simulink model "CLA_Sample"  (R2022b)
settings: Solver=FixedStepAuto  StartTime=0.0  StopTime=Inf  RelTol=1e-3  EnableMultiTasking=on
model workspace (MAT data in the model file):
  ADC_Gain = 1241.21212121
  DAC_Gain = 0.000805860805861
  Inductor_Current_Divider_Gain_Phase_A = 33.4
  Inductor_Current_Divider_Gain_Phase_B = 33.4
  Vbulk_Divider_Gain = 276.854928018
  Vin_Divider_Gain = 556.17352614
undefined symbols (not defined in the file or in its folder): GPTRIP1SEL, GPTRIP2SEL, SCI_A_Transmit, SCI_A_Transmit_Current_Suffix, SCI_A_Transmit_one_shot_Suffix, SCI_A_Transmit_Polarity_Suffix, SCI_A_Transmit_relay_Suffix, SCI_A_Transmit_Vbulk_Suffix, SCI_A_Transmit_Vin_rms_Suffix, SCI_A_Transmit_Vin_Suffix, SCI_A_Transmit_Vmid_Suffix, SCI_A_Transmit_Vp_Suffix, SCI_A_Transmit_Vpfc_Suffix, TZ1, TZ2
libraries: c280xlib x33, simulink x17, c2802xlib x15, c2000lib x1, c2806xlib x1
(part 5 of 5)

== system CLA_Sample/PWM Update @65KHz/Fixed Duty update_Phase_B/Archive/If Action Subsystem3/If Action Subsystem5 ==
  Action Port : ActionPort
  Constant : Constant  Value=100
  Data Store Read : DataStoreRead  DataStoreName=PWM_Duty_UART  IndexOptions=Index vector (dialog)  Indices=1  OutputSizes=1
  Data Store Read2 : DataStoreRead  DataStoreName=PWM_Duty_UART  IndexOptions=Index vector (dialog)  Indices=1  OutputSizes=1
  Data Store Read3 : DataStoreRead  DataStoreName=PFC_en_Phase_A  IndexOptions=Index vector (dialog)  Indices=1  OutputSizes=1
  Data Store Read4 : DataStoreRead  DataStoreName=One_Shot_Bar  IndexOptions=Index vector (dialog)  Indices=1  OutputSizes=1
  Data Store Write : DataStoreWrite  DataStoreName=PWM_DutyNearzero  IndexOptions=Index vector (dialog)  Indices=1  OutputSizes=1
  Product1 : Product  Inputs=3  OutDataTypeStr=double
  Subtract : Sum  Inputs=+-
  wires:
  Data Store Read4/1 -> Product1/2
  Data Store Read3/1 -> Product1/1
  Data Store Read2/1 -> Product1/3
  Constant/1 -> Subtract/1
  Data Store Read/1 -> Subtract/2
  Product1/1 -> Data Store Write/1

== system CLA_Sample/PWM Update @65KHz/Fixed Duty update_Phase_C/Archive/If Action Subsystem3/If Action Subsystem4 ==
  Action Port : ActionPort
  Data Store Read : DataStoreRead  DataStoreName=PWM_Duty_UART  IndexOptions=Index vector (dialog)  Indices=1  OutputSizes=1
  Data Store Read2 : DataStoreRead  DataStoreName=PWM_Duty_UART  IndexOptions=Index vector (dialog)  Indices=1  OutputSizes=1
  Data Store Read3 : DataStoreRead  DataStoreName=PFC_en_Phase_A  IndexOptions=Index vector (dialog)  Indices=1  OutputSizes=1
  Data Store Read4 : DataStoreRead  DataStoreName=One_Shot_Bar  IndexOptions=Index vector (dialog)  Indices=1  OutputSizes=1
  Data Store Write : DataStoreWrite  DataStoreName=PWM_DutyNearzero  IndexOptions=Index vector (dialog)  Indices=1  OutputSizes=1
  Product1 : Product  Inputs=3  OutDataTypeStr=double
  wires:
  Product1/1 -> Data Store Write/1
  Data Store Read3/1 -> Product1/1
  Data Store Read4/1 -> Product1/2
  Data Store Read2/1 -> Product1/3

== system CLA_Sample/PWM Update @65KHz/Fixed Duty update_Phase_C/Archive/If Action Subsystem3/If Action Subsystem5 ==
  Action Port : ActionPort
  Constant : Constant  Value=100
  Data Store Read : DataStoreRead  DataStoreName=PWM_Duty_UART  IndexOptions=Index vector (dialog)  Indices=1  OutputSizes=1
  Data Store Read2 : DataStoreRead  DataStoreName=PWM_Duty_UART  IndexOptions=Index vector (dialog)  Indices=1  OutputSizes=1
  Data Store Read3 : DataStoreRead  DataStoreName=PFC_en_Phase_A  IndexOptions=Index vector (dialog)  Indices=1  OutputSizes=1
  Data Store Read4 : DataStoreRead  DataStoreName=One_Shot_Bar  IndexOptions=Index vector (dialog)  Indices=1  OutputSizes=1
  Data Store Write : DataStoreWrite  DataStoreName=PWM_DutyNearzero  IndexOptions=Index vector (dialog)  Indices=1  OutputSizes=1
  Product1 : Product  Inputs=3  OutDataTypeStr=double
  Subtract : Sum  Inputs=+-
  wires:
  Data Store Read4/1 -> Product1/2
  Data Store Read3/1 -> Product1/1
  Data Store Read2/1 -> Product1/3
  Constant/1 -> Subtract/1
  Data Store Read/1 -> Subtract/2
  Product1/1 -> Data Store Write/1

== stateflow chart CLA_Sample/Calibration,RMS, Fault Protection @5kHz/Fault checking/If Action Subsystem/Phase_C_Fault/Fault Check (Input OVP)_Phase_C/Chart1 ==
  (default) -> (junction 2)
  (junction 2) -> (junction 81) [order 1] : [input > Voff_Threshold]
  (junction 81) -> (junction 82) : {
      | Input_OVP_Flag=1;
      | Voff_Threshold=95;
      | }
  (junction 2) -> (junction 84) [order 2] : {
      | Input_OVP_Flag=0;
      | Voff_Threshold = 100;
      | }
  (junction 82) -> (junction 84)
  data: input input double; Input_OVP_Flag output double =0; Voff_Threshold local =100

== stateflow chart CLA_Sample/Calibration,RMS, Fault Protection @5kHz/Fault checking/If Action Subsystem/Phase_C_Fault/Fault Check (Input UVP)_Phase_C/Chart1 ==
  (default) -> (junction 2)
  (junction 2) -> (junction 81) [order 1] : [input > Von_Threshold]
  (junction 81) -> (junction 82) : {
      | Input_UVP_Flag=0;
      | Von_Threshold=8;
      | }
  (junction 2) -> (junction 84) [order 2] : {
      | Input_UVP_Flag=1;
      | Von_Threshold = 12;
      | }
  (junction 82) -> (junction 84)
  data: input input double; Input_UVP_Flag output double =1; Von_Threshold local =12

== stateflow chart CLA_Sample/Calibration,RMS, Fault Protection @5kHz/Fault checking/If Action Subsystem/Phase_C_Fault/Input current_OCP_Phase_C/Chart2 ==
  note: Input_in > 1A, Iin_OCP_Flag=1.
  (default) -> (junction 2)
  (junction 2) -> (junction 81) [order 1] : [input_Iin > OCP_Threshold]
  (junction 81) -> (junction 82) : {Iin_OCP_Flag=1;
      | OCP_Threshold=14;
      | }
  (junction 2) -> (junction 84) [order 2] : {Iin_OCP_Flag=0;
      | OCP_Threshold=15;}
  (junction 82) -> (junction 84)
  data: input_Iin input double; Iin_OCP_Flag output double =1; data local; OCP_Threshold input; OCP_Threshold output

== stateflow chart CLA_Sample/Calibration,RMS, Fault Protection @5kHz/Fault checking/If Action Subsystem/PFC_en_update_Phase_C/Chart ==
  note: Local variables
      | VbusRefTemp
      | SoftStartCnt
  note: Verror = Vbulk_Ref_ADC_adjusted - Vbulk_ADC;
  (default) -> (junction 47)
  (junction 47) -> (junction 50) [order 4]
  (junction 47) -> (junction 68) [order 1] : [Vin_OVP_Flag]
  (junction 68) -> (junction 80) : {PFC_en=0;}
  (junction 47) -> (junction 15) [order 2] : [Iin_OCP_Flag]
  (junction 50) -> (junction 52) : {
      | PFC_en=1;
      | PFC_en1=1;
      | }
  (junction 47) -> (junction 5) [order 3] : [Vin_UVP_Flag]
  (junction 80) -> (junction 82)
  (junction 82) -> (junction 84)
  (junction 5) -> (junction 38) : {
      | PFC_en=0;
      | PFC_en1=0;
      | }
  (junction 15) -> (junction 20) : {PFC_en=0;
      | PFC_en1=0;}
  (junction 52) -> (junction 38)
  (junction 20) -> (junction 38)
  (junction 84) -> (junction 20)
  data: Vin_UVP_Flag input; VbusRefTemp local =0; Vin_OVP_Flag input; SoftStartCnt local =0; Vbulk_Ref_ADC_Hard_Value local =0; UVPCnt local =0; PFC_en output; PFC_en1 output; Iin_OCP_Flag input; Iin_OCP_Flag1 local

== stateflow chart CLA_Sample/Calibration,RMS, Fault Protection @5kHz/Polarity & Near Zero check/Polarity_Near_zero_Phase_C/Chart ==
  note: 1-> Polarity -> Positive Half cycle
      | 0-> Polarity -> Negative Half cycle
  (default) -> (junction 89) : {Vabs=abs(input);}
  (junction 89) -> (junction 99) [order 1] : [input>Vref]
  (junction 89) -> (junction 103) [order 2] : {Polarity=0;}
  (junction 99) -> (junction 101) : {Polarity=1;}
  (junction 103) -> (junction 142) [order 3]
  (junction 101) -> (junction 103)
  (junction 103) -> (junction 133) [order 1] : [Near_zero==0]
      | {Count = Count+1;}
  (junction 142) -> (junction 146)
  (junction 103) -> (junction 120) [order 2] : [Vabs<VZCD_Gap]
      | {Near_zero=0;}
  (junction 133) -> (junction 120) [order 2]
  (junction 133) -> (junction 136) [order 1] : [Count>10]
      | {Near_zero=1;
      | Count=0;}
  (junction 146) -> (junction 120)
  (junction 136) -> (junction 120)
  data: input input double; Polarity output; Vabs local double =0; Vref input; VZCD_Gap input; Near_zero output double =0; Count local =0

== stateflow chart CLA_Sample/Calibration,RMS, Fault Protection @5kHz/Voltage RMS//Averag Calculation/Phase_C/RMS Current Calculation_Phase_C/Chart ==
  note: counter > (0.5 / minimum line frequncy) x execution frequency of this loop
      | = [ 1 / (2 x 47 Hz) ] x 5 kHz = 53.191
      | Minimum frequency detection is 47Hz.
      | This can detect the voltage change in ~10.63 ms (max).
  (default) -> (junction 2) : {Vabs=abs(input);}
  (junction 2) -> (junction 81) [order 1] : [Vabs>max_tmp]
  (junction 81) -> (junction 82) : {
      | max_tmp=Vabs;
      | counter=counter+1;
      | timer=timer+1;
      | }
  (junction 2) -> (junction 84) [order 2] : {
      | counter=counter+1;
      | timer=timer+1;
      | }
  (junction 82) -> (junction 84)
  (junction 84) -> (junction 8)
  (junction 8) -> (junction 71) [order 1] : [counter==53]
  (junction 71) -> (junction 72) : {
      | counter=0;
      | Vpeak=max_tmp;
      | Vrms = 0.7071*Vpeak;
      | max_tmp=0;
      | }
  (junction 8) -> (junction 64) [order 2]
  (junction 72) -> (junction 64)
  data: input input double; max_tmp local double =0; counter local double =0; Vpeak output; Vrms output; timer local double =0; Vabs local double =0

== stateflow chart CLA_Sample/Calibration,RMS, Fault Protection @5kHz/Voltage RMS//Averag Calculation/Phase_A/RMS Current Calculation_Phase_A/Chart ==
  note: counter > (0.5 / minimum line frequncy) x execution frequency of this loop
      | = [ 1 / (2 x 47 Hz) ] x 5 kHz = 53.191
      | Minimum frequency detection is 47Hz.
      | This can detect the voltage change in ~10.63 ms (max).
  (default) -> (junction 2) : {Vabs=abs(input);}
  (junction 2) -> (junction 81) [order 1] : [Vabs>max_tmp]
  (junction 81) -> (junction 82) : {
      | max_tmp=Vabs;
      | counter=counter+1;
      | timer=timer+1;
      | }
  (junction 2) -> (junction 84) [order 2] : {
      | counter=counter+1;
      | timer=timer+1;
      | }
  (junction 82) -> (junction 84)
  (junction 84) -> (junction 8)
  (junction 8) -> (junction 71) [order 1] : [counter==53]
  (junction 71) -> (junction 72) : {
      | counter=0;
      | Vpeak=max_tmp;
      | Vrms = 0.7071*Vpeak;
      | max_tmp=0;
      | }
  (junction 8) -> (junction 64) [order 2]
  (junction 72) -> (junction 64)
  data: input input double; max_tmp local double =0; counter local double =0; Vpeak output; Vrms output; timer local double =0; Vabs local double =0

== stateflow chart CLA_Sample/Calibration,RMS, Fault Protection @5kHz/Voltage RMS//Averag Calculation/Phase_B/RMS Current Calculation_Phase_B/Chart ==
  note: counter > (0.5 / minimum line frequncy) x execution frequency of this loop
      | = [ 1 / (2 x 47 Hz) ] x 5 kHz = 53.191
      | Minimum frequency detection is 47Hz.
      | This can detect the voltage change in ~10.63 ms (max).
  (default) -> (junction 2) : {Vabs=abs(input);}
  (junction 2) -> (junction 81) [order 1] : [Vabs>max_tmp]
  (junction 81) -> (junction 82) : {
      | max_tmp=Vabs;
      | counter=counter+1;
      | timer=timer+1;
      | }
  (junction 2) -> (junction 84) [order 2] : {
      | counter=counter+1;
      | timer=timer+1;
      | }
  (junction 82) -> (junction 84)
  (junction 84) -> (junction 8)
  (junction 8) -> (junction 71) [order 1] : [counter==53]
  (junction 71) -> (junction 72) : {
      | counter=0;
      | Vpeak=max_tmp;
      | Vrms = 0.7071*Vpeak;
      | max_tmp=0;
      | }
  (junction 8) -> (junction 64) [order 2]
  (junction 72) -> (junction 64)
  data: input input double; max_tmp local double =0; counter local double =0; Vpeak output; Vrms output; timer local double =0; Vabs local double =0

== stateflow chart CLA_Sample/PWM Update @65KHz/Closed loop PWM generation (Control)/If Action Subsystem/Function-Call Subsystem/Chart4 ==
  (default) -> (junction 18) : {
      | output_y = b0*input_u + b1*input_z1 + b2*input_z2 - a1*output_z1 - a2*output_z2;
      |
      | }
  (junction 18) -> (junction 23) [commented out]
  (junction 18) -> (junction 15) [order 2]
  (junction 18) -> (junction 15) [order 1] : [output_y>Max_Duty]{output_y=Max_Duty;}
  (junction 23) -> (junction 27) [commented out] : [output_y<23]
      |
      | {
      | output_y=0;
      | }
  (junction 27) -> (junction 15) [commented out]
  (junction 15) -> (junction 16) : {
      | input_z2 = input_z1;
      | input_z1 = input_u;
      | output_z2 = output_z1;
      | output_z1 = output_y;}
  (junction 16) -> (junction 31) [order 2]
  (junction 16) -> (junction 31) [order 1] : [output_y<45]
      | {
      | output_y=0;
      | }
  data: Max_Duty input; input_z2 local =0; input_z1 local =0; output_z2 local =0; output_z1 local =0; output_y output; input_u input; b0 input; b1 input; b2 input; a1 input; a2 input

== stateflow chart CLA_Sample/Calibration,RMS, Fault Protection @5kHz/Calibration/Calibration_3phase/Chart ==
  note: Local variables
      | VbusRefTemp
      | SoftStartCnt
  note: Verror = Vbulk_Ref_ADC_adjusted - Vbulk_ADC;
  (default) -> (junction 47)
  (junction 47) -> (junction 50) [order 4]
  (junction 47) -> (junction 68) [order 1] : [~Calibration_Done_Phase_C]
  (junction 68) -> (junction 80) : {Calibration_Done=0;}
  (junction 47) -> (junction 15) [order 2] : [~Calibration_Done_Phase_B]
  (junction 50) -> (junction 52) : {
      | Calibration_Done=1;
      | }
  (junction 47) -> (junction 5) [order 3] : [~Calibration_Done_Phase_A]
  (junction 80) -> (junction 82)
  (junction 82) -> (junction 84)
  (junction 5) -> (junction 38) : {
      | Calibration_Done=0;
      | }
  (junction 15) -> (junction 20) : {Calibration_Done=0;}
  (junction 52) -> (junction 38)
  (junction 20) -> (junction 38)
  (junction 84) -> (junction 20)
  data: Calibration_Done_Phase_A input; Calibration_Done_Phase_B input; VbusRefTemp local =0; SoftStartCnt local =0; Vbulk_Ref_ADC_Hard_Value local =0; UVPCnt local =0; Calibration_Done output; Calibration_Done_Phase_C input; Iin_OCP_Flag1 local

== stateflow chart CLA_Sample/Calibration,RMS, Fault Protection @5kHz/Fault checking/If Action Subsystem/Output Voltage_Latch_OVP/Chart2 ==
  note: "One_Shot_Bar = 0" means fault occurs and turn off switching.
  (default) -> (junction 2)
  (junction 2) -> (junction 81) [order 1] : [input_Vbulk > Vbulk_OVP_Threshold]
  (junction 81) -> (junction 82) : {
      | One_Shot_Bar=0;
      | }
  (junction 2) -> (junction 84) [order 2]
  (junction 82) -> (junction 84)
  data: input_Vbulk input double; One_Shot_Bar output double =1; Vbulk_OVP_Threshold input

== matlab function CLA_Sample/UART reporting @ 1Hz/SCI_A_Transmit_function/MATLAB Function ==
  data: Main_number input; Digit_5 output; Divider input; Digit_4 output; Digit_3 output; Digit_2 output; Digit_1 output
function [Digit_5,Digit_4,Digit_3,Digit_2,Digit_1]  = fcn(Main_number,Divider)

R_Digit_5 = rem(Main_number,Divider);
Q_Digit_5 = (Main_number-R_Digit_5)/Divider;
Digit_5 = uint8(Q_Digit_5);
%Digit_5 done

R_Digit_4 = rem(R_Digit_5,Divider/10);
Q_Digit_4 = (R_Digit_5-R_Digit_4)/(Divider/10);
Digit_4 = uint8(Q_Digit_4);
%Digit_4 done

R_Digit_3 = rem(R_Digit_4,Divider/100);
Q_Digit_3 = (R_Digit_4-R_Digit_3)/(Divider/100);
Digit_3 = uint8(Q_Digit_3);
%Digit_3 done

R_Digit_2 = rem(R_Digit_3,Divider/1000);
Q_Digit_2 = (R_Digit_3-R_Digit_2)/(Divider/1000);
Digit_2 = uint8(Q_Digit_2);
%Digit_2 done

R_Digit_1 = rem(R_Digit_2,Divider/10000);
Q_Digit_1 = (R_Digit_2-R_Digit_1)/(Divider/10000);
Digit_1 = uint8(Q_Digit_1);
%Digit_1 done
end

== stateflow chart CLA_Sample/Calibration,RMS, Fault Protection @5kHz/Voltage RMS//Averag Calculation/Phase_A/RMS Voltage Calculation_Phase_A/Chart ==
  note: counter > (0.5 / minimum line frequncy) x execution frequency of this loop
      | = [ 1 / (2 x 47 Hz) ] x 5 kHz = 53.191
      | Minimum frequency detection is 47Hz.
      | This can detect the voltage change in ~10.63 ms (max).
  (default) -> (junction 2) : {Vabs=abs(input);}
  (junction 2) -> (junction 81) [order 1] : [Vabs>max_tmp]
  (junction 81) -> (junction 82) : {
      | max_tmp=Vabs;
      | counter=counter+1;
      | timer=timer+1;
      | }
  (junction 2) -> (junction 84) [order 2] : {
      | counter=counter+1;
      | timer=timer+1;
      | }
  (junction 82) -> (junction 84)
  (junction 84) -> (junction 8)
  (junction 8) -> (junction 71) [order 1] : [counter==53]
  (junction 71) -> (junction 72) : {
      | counter=0;
      | Vpeak=max_tmp;
      | Vrms = 0.7071*Vpeak;
      | max_tmp=0;
      | }
  (junction 8) -> (junction 64) [order 2]
  (junction 72) -> (junction 64)
  data: input input double; max_tmp local double =0; counter local double =0; Vpeak output; Vrms output; timer local double =0; Vabs local double =0

== stateflow chart CLA_Sample/Calibration,RMS, Fault Protection @5kHz/Fault checking/If Action Subsystem/Phase_A_Fault/Fault Check (Input UVP)_Phase_A /Chart1 ==
  (default) -> (junction 2)
  (junction 2) -> (junction 81) [order 1] : [input > Von_Threshold]
  (junction 81) -> (junction 82) : {
      | Input_UVP_Flag=0;
      | Von_Threshold=8;
      | }
  (junction 2) -> (junction 84) [order 2] : {
      | Input_UVP_Flag=1;
      | Von_Threshold = 12;
      | }
  (junction 82) -> (junction 84)
  data: input input double; Input_UVP_Flag output double =1; Von_Threshold local =12

== stateflow chart CLA_Sample/Calibration,RMS, Fault Protection @5kHz/Polarity & Near Zero check/Polarity_Near_zero_Phase_A/Chart ==
  note: 1-> Polarity -> Positive Half cycle
      | 0-> Polarity -> Negative Half cycle
  (default) -> (junction 89) : {Vabs=abs(input);}
  (junction 89) -> (junction 99) [order 1] : [input>Vref]
  (junction 89) -> (junction 103) [order 2] : {Polarity=0;}
  (junction 99) -> (junction 101) : {Polarity=1;}
  (junction 103) -> (junction 142) [order 3]
  (junction 101) -> (junction 103)
  (junction 103) -> (junction 133) [order 1] : [Near_zero==0]
      | {Count = Count+1;}
  (junction 142) -> (junction 146)
  (junction 103) -> (junction 120) [order 2] : [Vabs<VZCD_Gap]
      | {Near_zero=0;}
  (junction 133) -> (junction 120) [order 2]
  (junction 133) -> (junction 136) [order 1] : [Count>10]
      | {Near_zero=1;
      | Count=0;}
  (junction 146) -> (junction 120)
  (junction 136) -> (junction 120)
  data: input input double; Polarity output; Vabs local double =0; Vref input; VZCD_Gap input; Near_zero output double =0; Count local =0

== stateflow chart CLA_Sample/Calibration,RMS, Fault Protection @5kHz/Relay control/Subsystem/Relay_Control1 ==
  (default) -> (junction 10)
  (junction 10) -> (junction 37) [order 2]
  (junction 37) -> (junction 40) [order 2]
  (junction 10) -> (junction 12) [order 1] : [Vin_peak_ADC>Relay_TurnON_Threshold_ADC]
  (junction 37) -> (junction 25) [order 1] : [Vin_peak_ADC<(Relay_TurnON_Threshold_ADC-5)]
  (junction 40) -> (junction 42)
  (junction 12) -> (junction 49) [order 2] : %% Relay has started.
  (junction 49) -> (junction 67) [order 1] : [PWM_Turned_on==0]
  (junction 67) -> (junction 79) [order 2]
  (junction 12) -> (junction 19) [order 1] : [Relay_Started==0]
      | {Relay_Start_Count = Relay_Start_Count + 1;}
  (junction 49) -> (junction 73) [order 2]
  (junction 67) -> (junction 68) [order 1] : [Counter_Relay > 400]
      | {
      | PWM_Turned_on=1;
      | Counter_Relay=0;
      | }
  (junction 79) -> (junction 81) : {
      | Counter_Relay = Counter_Relay + 1;
      | PWM_Turned_on=0;
      | }
  (junction 25) -> (junction 27) : [PFC_en==0]
      | {
      | Relay_Started=0;
      | Relay_Start_Count = 0;
      | PWM_Turned_on=0;
      | %% Turn off relay GPIO here
      | }
  (junction 19) -> (junction 54) [order 2]
  (junction 19) -> (junction 21) [order 1] : %%[((Vin_peak_ADC-(Vbulk_ADC_Average/2))<VIN_VBUS_DIFF)]
      | %% Vbulk is within range
  (junction 54) -> (junction 51)
  (junction 21) -> (junction 23) : [Relay_Start_Count > RELAY_START_DELAY]
      | %% waited long enough....
      |
      | {
      | Relay_Start_Count = 0;
      | Relay_Started = 1;
      | Counter_Relay=0;
      | %% Start relay GPIO here
      | }
      |
      | %% Relay started
  (junction 23) -> (junction 51)
  (junction 51) -> (junction 73)
  (junction 73) -> (junction 68)
  (junction 81) -> (junction 68)
  (junction 27) -> (junction 81)
  (junction 42) -> (junction 27)
  data: Vin_peak_ADC input; Relay_TurnON_Threshold_ADC input; RELAY_START_DELAY input; Vbulk_ADC_Average input; Relay_Start_Count local double =0; VIN_VBUS_DIFF input; PFC_en input; Relay_Started output =0; PWM_Turned_on output double =0; Counter_Relay local =0

== stateflow chart CLA_Sample/Calibration,RMS, Fault Protection @5kHz/Voltage RMS//Averag Calculation/Phase_A/Vin_ADC Averaging_Phase_A/Chart1 ==
  (default) -> (junction 1) : {
      | output_y = b0*input_u + b1*input_z1 - a1*output_z1;
      | input_z1 = input_u;
      | output_z1 = output_y;
      | }
  data: input_z1 local =0; output_z1 local =0; output_y output; input_u input; b0 input; b1 input; a1 input

== stateflow chart CLA_Sample/Calibration,RMS, Fault Protection @5kHz/Calibration/Chart ==
  note: For DC Mode
      | Ensure Polarity does not change for e.g, 100 cycles. Before executing the loop
  note: Add more signals if required.
  (default) -> (junction 4)
  (junction 22) -> (junction 45) [order 2]
  (junction 35) -> (junction 22) [order 2]
  (junction 4) -> (junction 10) [order 1]
  (junction 4) -> (junction 50) [order 3]
  (junction 50) -> (junction 56) [order 2]
  (junction 56) -> (junction 62) [order 1]
  (junction 62) -> (junction 35) [order 1]
  (junction 4) -> (junction 20) [order 2] : [Polarity_z1~=Polarity]
      |
      | {
      | Local_AC_Cycles_Count = Local_AC_Cycles_Count + 1;
      | }
  (junction 22) -> (junction 24) [order 1] : [Local_AC_Cycles_Count==AC_Cycles ]
      | {
      | output_signal_1=input_signal_1_sum/Local_counter;
      | output_signal_2=input_signal_2_sum/Local_counter;
      | Calibration_Done=1;
      | }
  (junction 45) -> (junction 47)
  (junction 56) -> (junction 60) [order 2] : [Local_DC_Cycles_Count>=125]
      |
      | {input_signal_1_sum=input_signal_1+input_signal_1_sum;
      |
      | Local_counter_DC = Local_counter_DC + 1;
      | }
  (junction 50) -> (junction 53) [order 1] : [Polarity_z1==Polarity]
      |
      | {
      | Local_DC_Cycles_Count = Local_DC_Cycles_Count + 1;
      | }
  (junction 35) -> (junction 37) [order 1] : [(Local_AC_Cycles_Count>0) && (Local_AC_Cycles_Count<AC_Cycles)]
      | {input_signal_1_sum=input_signal_1+input_signal_1_sum;
      | input_signal_2_sum=input_signal_2+input_signal_2_sum;
      | Local_counter = Local_counter + 1;}
  (junction 10) -> (junction 17) : [Calibration_Done==1]
  (junction 62) -> (junction 64) [order 2] : [Local_counter_DC>=10000]
      |
      | {output_signal_1=input_signal_1_sum/Local_counter_DC;
      |
      | Calibration_Done=1;
      | }
  (junction 47) -> (junction 24)
  (junction 24) -> (junction 37)
  (junction 17) -> (junction 20)
  (junction 53) -> (junction 20)
  (junction 60) -> (junction 53)
  (junction 64) -> (junction 60)
  (junction 37) -> (junction 64)
  data: Polarity_z1 input; Calibration_Done input; Polarity input; input_signal_1 input; input_signal_2 input; AC_Cycles input; Local_counter local double =1; input_signal_1_sum local =0; input_signal_2_sum local =0; output_signal_1 output; output_signal_2 output; Calibration_Done output; Local_AC_Cycles_Count local double =0; Local_DC_Cycles_Count local =0; Local_counter_DC local =0

== stateflow chart CLA_Sample/Calibration,RMS, Fault Protection @5kHz/Calibration/Calibration_Phase_C/Chart1 ==
  note: Add more signals if required.
  (default) -> (junction 4)
  (junction 4) -> (junction 10) [order 1]
  (junction 4) -> (junction 22) [order 3]
  (junction 10) -> (junction 17) : [Calibration_Done==1]
  (junction 4) -> (junction 20) [order 2] : [Local_counter<Counter_for_calibration]
      |
      | {
      |
      | input_signal_1_sum=input_signal_1+input_signal_1_sum;
      | input_signal_2_sum=input_signal_2+input_signal_2_sum;
      | Local_counter = Local_counter + 1;
      |
      | }
  (junction 22) -> (junction 24) : %% Local_counter==Counter_for_calibration
      | %% Meaning that count is completed.
      |
      |
      | {
      | output_signal_1=input_signal_1_sum/Local_counter;
      | output_signal_2=input_signal_2_sum/Local_counter;
      | Calibration_Done=1;
      |
      | Local_counter=0; %% Not required, but do it anyway.
      | }
  (junction 17) -> (junction 20)
  (junction 20) -> (junction 24)
  data: Calibration_Done input; input_signal_1 input; input_signal_2 input; Counter_for_calibration input; Local_counter local double =0; input_signal_1_sum local =0; input_signal_2_sum local =0; output_signal_1 output; output_signal_2 output; Calibration_Done output

== stateflow chart CLA_Sample/Calibration,RMS, Fault Protection @5kHz/Voltage RMS//Averag Calculation/Vbulk_ADC Averaging/Chart1 ==
  (default) -> (junction 1) : {
      | output_y = b0*input_u + b1*input_z1 - a1*output_z1;
      | input_z1 = input_u;
      | output_z1 = output_y;
      | }
  data: input_z1 local =0; output_z1 local =0; output_y output; input_u input; b0 input; b1 input; a1 input

== stateflow chart CLA_Sample/Calibration,RMS, Fault Protection @5kHz/Voltage RMS//Averag Calculation/Phase_C/RMS Voltage Calculation_Phase_C/Chart ==
  note: counter > (0.5 / minimum line frequncy) x execution frequency of this loop
      | = [ 1 / (2 x 47 Hz) ] x 5 kHz = 53.191
      | Minimum frequency detection is 47Hz.
      | This can detect the voltage change in ~10.63 ms (max).
  (default) -> (junction 2) : {Vabs=abs(input);}
  (junction 2) -> (junction 81) [order 1] : [Vabs>max_tmp]
  (junction 81) -> (junction 82) : {
      | max_tmp=Vabs;
      | counter=counter+1;
      | timer=timer+1;
      | }
  (junction 2) -> (junction 84) [order 2] : {
      | counter=counter+1;
      | timer=timer+1;
      | }
  (junction 82) -> (junction 84)
  (junction 84) -> (junction 8)
  (junction 8) -> (junction 71) [order 1] : [counter==53]
  (junction 71) -> (junction 72) : {
      | counter=0;
      | Vpeak=max_tmp;
      | Vrms = 0.7071*Vpeak;
      | max_tmp=0;
      | }
  (junction 8) -> (junction 64) [order 2]
  (junction 72) -> (junction 64)
  data: input input double; max_tmp local double =0; counter local double =0; Vpeak output; Vrms output; timer local double =0; Vabs local double =0

== stateflow chart CLA_Sample/Calibration,RMS, Fault Protection @5kHz/Voltage RMS//Averag Calculation/Phase_C/Vin_ADC Averaging_Phase_C/Chart1 ==
  (default) -> (junction 1) : {
      | output_y = b0*input_u + b1*input_z1 - a1*output_z1;
      | input_z1 = input_u;
      | output_z1 = output_y;
      | }
  data: input_z1 local =0; output_z1 local =0; output_y output; input_u input; b0 input; b1 input; a1 input

== stateflow chart CLA_Sample/Calibration,RMS, Fault Protection @5kHz/Soft Start/Chart ==
  note: Verror = Vbulk_Ref_ADC_adjusted - Vbulk_ADC;
  note: Local variables
      | VbusRefTemp
      | SoftStartCnt
  (default) -> (junction 47)
  (junction 47) -> (junction 50) [order 2]
  (junction 50) -> (junction 52) : {
      | First_Pass=1;
      | Soft_Start=1;
      | SoftStartCnt=1;
      | Debug=1;
      | }
  (junction 47) -> (junction 5) [order 1] : [PFC_en & Relay_started]
  (junction 5) -> (junction 7) [order 1] : [First_Pass]
  (junction 5) -> (junction 15) [order 2] : [Soft_Start]
  (junction 15) -> (junction 18) [order 1] : [SoftStartCnt>100]
      | %% At every 5 cycles (total 1ms),
  (junction 18) -> (junction 23) [order 2] : {Debug=Vbulk_Ref_ADC_adjusted;}
  (junction 23) -> (junction 31) [order 2] : {Debug=6;}
  (junction 31) -> (junction 55) [order 1] : [abs(Vbulk_Ref_ADC_adjusted - Vbulk_Ref_ADC)<5]
  (junction 7) -> (junction 10) : {
      | Vbulk_Ref_ADC_adjusted = Vbulk_ADC;
      | %Vbulk_Ref_ADC_adjusted = Vbulk_Ref_ADC;
      | First_Pass = 0;
      | Debug=2;
      |
      | }
  (junction 5) -> (junction 38) [order 3] : {
      | Debug=3;
      | %Vbulk_Ref_ADC_adjusted=Vbulk_Ref_ADC;
      | }
  (junction 15) -> (junction 20) [order 2] : {SoftStartCnt = SoftStartCnt + 1;
      | Debug=4;}
      | %% incerase the counter first.
  (junction 18) -> (junction 64) [order 1] : [Vbulk_Ref_ADC_adjusted < Vbulk_Ref_ADC]
      | {Vbulk_Ref_ADC_adjusted = Vbulk_Ref_ADC_adjusted + 1;}
      | %% Increase the reference voltage
  (junction 23) -> (junction 26) [order 1] : [Vbulk_Ref_ADC_adjusted > Vbulk_Ref_ADC]
      | {Vbulk_Ref_ADC_adjusted = Vbulk_Ref_ADC_adjusted - 1;
      | }
      | %% Reduce the reference voltage
  (junction 31) -> (junction 33) [order 2] : {Soft_Start=0;
      | SoftStartCnt=0;
      | Debug=7;}
      | %% End soft start
  (junction 55) -> (junction 57) : {Soft_Start=0;
      | SoftStartCnt=0;
      | Vbulk_Ref_ADC_adjusted=Vbulk_Ref_ADC;
      | Debug=8;}
  (junction 64) -> (junction 28) [order 2]
  (junction 64) -> (junction 28) [order 1] : [Vbulk_Ref_ADC_adjusted < Vbulk_ADC]
      | {Vbulk_Ref_ADC_adjusted = Vbulk_ADC ;}
      | %% Increase the reference voltage
  (junction 52) -> (junction 10)
  (junction 10) -> (junction 38)
  (junction 26) -> (junction 28)
  (junction 33) -> (junction 26)
  (junction 57) -> (junction 33)
  (junction 20) -> (junction 38)
  (junction 28) -> (junction 20)
  data: Relay_started input; Debug output; PFC_en input; Vbulk_ADC input; First_Pass input; VbusRefTemp local =0; First_Pass output; Soft_Start output; Soft_Start input; SoftStartCnt local =0; Vbulk_Ref_ADC input; Vbulk_Ref_ADC_adjusted output; Vbulk_Ref_ADC_Hard_Value local =0; First_Pass1 local

== stateflow chart CLA_Sample/Calibration,RMS, Fault Protection @5kHz/Fault checking/If Action Subsystem/PFC_en_update_3Phase/Chart ==
  note: Local variables
      | VbusRefTemp
      | SoftStartCnt
  note: Verror = Vbulk_Ref_ADC_adjusted - Vbulk_ADC;
  (default) -> (junction 47)
  (junction 47) -> (junction 50) [order 4]
  (junction 47) -> (junction 68) [order 1] : [~PFC_en_Phase_C]
  (junction 68) -> (junction 80) : {PFC_en=0;}
  (junction 47) -> (junction 15) [order 2] : [~PFC_en_Phase_B]
  (junction 50) -> (junction 52) : {
      | PFC_en=1;
      | }
  (junction 47) -> (junction 5) [order 3] : [~PFC_en_Phase_A]
  (junction 80) -> (junction 82)
  (junction 82) -> (junction 84)
  (junction 5) -> (junction 38) : {
      | PFC_en=0;
      | }
  (junction 15) -> (junction 20) : {PFC_en=0;}
  (junction 52) -> (junction 38)
  (junction 20) -> (junction 38)
  (junction 84) -> (junction 20)
  data: PFC_en_Phase_A input; PFC_en_Phase_B input; VbusRefTemp local =0; SoftStartCnt local =0; Vbulk_Ref_ADC_Hard_Value local =0; UVPCnt local =0; PFC_en output; PFC_en_Phase_C input; Iin_OCP_Flag1 local

== stateflow chart CLA_Sample/Calibration,RMS, Fault Protection @5kHz/Calibration/Calibration_Phase_A/Chart1 ==
  note: Add more signals if required.
  (default) -> (junction 4)
  (junction 4) -> (junction 10) [order 1]
  (junction 4) -> (junction 22) [order 3]
  (junction 10) -> (junction 17) : [Calibration_Done==1]
  (junction 4) -> (junction 20) [order 2] : [Local_counter<Counter_for_calibration]
      |
      | {
      |
      | input_signal_1_sum=input_signal_1+input_signal_1_sum;
      | input_signal_2_sum=input_signal_2+input_signal_2_sum;
      | Local_counter = Local_counter + 1;
      |
      | }
  (junction 22) -> (junction 24) : %% Local_counter==Counter_for_calibration
      | %% Meaning that count is completed.
      |
      |
      | {
      | output_signal_1=input_signal_1_sum/Local_counter;
      | output_signal_2=input_signal_2_sum/Local_counter;
      | Calibration_Done=1;
      |
      | Local_counter=0; %% Not required, but do it anyway.
      | }
  (junction 17) -> (junction 20)
  (junction 20) -> (junction 24)
  data: Calibration_Done input; input_signal_1 input; input_signal_2 input; Counter_for_calibration input; Local_counter local double =0; input_signal_1_sum local =0; input_signal_2_sum local =0; output_signal_1 output; output_signal_2 output; Calibration_Done output

== stateflow chart CLA_Sample/PWM Update @65KHz/Closed loop PWM generation (Control)/If Action Subsystem/Function-Call Subsystem/Chart3 ==
  (default) -> (junction 18) : {
      | output_y = b0*input_u + b1*input_z1 + b2*input_z2 - a1*output_z1 - a2*output_z2;
      |
      | }
  (junction 18) -> (junction 23) [commented out]
  (junction 18) -> (junction 15) [order 2]
  (junction 18) -> (junction 15) [order 1] : [output_y>Max_Duty]{output_y=Max_Duty;}
  (junction 23) -> (junction 27) [commented out] : [output_y<23]
      |
      | {
      | output_y=0;
      | }
  (junction 27) -> (junction 15) [commented out]
  (junction 15) -> (junction 16) : {
      | input_z2 = input_z1;
      | input_z1 = input_u;
      | output_z2 = output_z1;
      | output_z1 = output_y;}
  (junction 16) -> (junction 31) [order 2]
  (junction 16) -> (junction 31) [order 1] : [output_y<45]
      | {
      | output_y=0;
      | }
  data: Max_Duty input; input_z2 local =0; input_z1 local =0; output_z2 local =0; output_z1 local =0; output_y output; input_u input; b0 input; b1 input; b2 input; a1 input; a2 input

== stateflow chart CLA_Sample/PWM Update @65KHz/Closed loop PWM generation (Control)/If Action Subsystem/Function-Call Subsystem/Chart1 ==
  (default) -> (junction 1) : {
      | output_y = b0*input_u + b1*input_z1 + b2*input_z2 - a1*output_z1 - a2*output_z2;
      | }
  (junction 1) -> (junction 21) [order 2]
  (junction 1) -> (junction 26) [commented out] : [output_y<23]{output_y=0;}
  (junction 21) -> (junction 23)
  (junction 1) -> (junction 15) [order 1] : [output_y>Max_Duty]{output_y=Max_Duty;}
  (junction 26) -> (junction 27) [commented out]
  (junction 23) -> (junction 15)
  (junction 27) -> (junction 15) [commented out]
  (junction 15) -> (junction 17) : {
      | input_z2 = input_z1;
      | input_z1 = input_u;
      | output_z2 = output_z1;
      | output_z1 = output_y;}
  data: Max_Duty input; input_z2 local =0; input_z1 local =0; output_z2 local =0; output_z1 local =0; output_y output; input_u input; b0 input; b1 input; b2 input; a1 input; a2 input

== stateflow chart CLA_Sample/PWM Update @65KHz/Closed loop PWM generation (Control)/If Action Subsystem/Function-Call Subsystem/Chart2 ==
  (default) -> (junction 18) : {
      | output_y = b0*input_u + b1*input_z1 + b2*input_z2 - a1*output_z1 - a2*output_z2;
      |
      | }
  (junction 18) -> (junction 23) [commented out]
  (junction 18) -> (junction 15) [order 2]
  (junction 18) -> (junction 15) [order 1] : [output_y>Max_Duty]{output_y=Max_Duty;}
  (junction 23) -> (junction 27) [commented out] : [output_y<23]
      |
      | {
      | output_y=0;
      | }
  (junction 27) -> (junction 15) [commented out]
  (junction 15) -> (junction 16) : {
      | input_z2 = input_z1;
      | input_z1 = input_u;
      | output_z2 = output_z1;
      | output_z1 = output_y;}
  (junction 16) -> (junction 31) [order 2]
  (junction 16) -> (junction 31) [order 1] : [output_y<45]
      | {
      | output_y=0;
      | }
  data: Max_Duty input; input_z2 local =0; input_z1 local =0; output_z2 local =0; output_z1 local =0; output_y output; input_u input; b0 input; b1 input; b2 input; a1 input; a2 input

== stateflow chart CLA_Sample/Calibration,RMS, Fault Protection @5kHz/Fault checking/If Action Subsystem/Phase_A_Fault/Input current_OCP_Phase_A/Chart2 ==
  note: Input_in > 1A, Iin_OCP_Flag=1.
  (default) -> (junction 2)
  (junction 2) -> (junction 81) [order 1] : [input_Iin > OCP_Threshold]
  (junction 81) -> (junction 82) : {Iin_OCP_Flag=1;
      | OCP_Threshold=14;
      | }
  (junction 2) -> (junction 84) [order 2] : {Iin_OCP_Flag=0;
      | OCP_Threshold=15;}
  (junction 82) -> (junction 84)
  data: input_Iin input double; Iin_OCP_Flag output double =1; data local; Iin_OCP_Threshold local double =10; OCP_Threshold input; OCP_Threshold output

== stateflow chart CLA_Sample/Calibration,RMS, Fault Protection @5kHz/Fault checking/If Action Subsystem/Phase_A_Fault/Fault Check (Input OVP)_Phase_A /Chart1 ==
  (default) -> (junction 2)
  (junction 2) -> (junction 81) [order 1] : [input > Voff_Threshold]
  (junction 81) -> (junction 82) : {
      | Input_OVP_Flag=1;
      | Voff_Threshold=95;
      | }
  (junction 2) -> (junction 84) [order 2] : {
      | Input_OVP_Flag=0;
      | Voff_Threshold = 100;
      | }
  (junction 82) -> (junction 84)
  data: input input double; Input_OVP_Flag output double =0; Voff_Threshold local =100

== stateflow chart CLA_Sample/Calibration,RMS, Fault Protection @5kHz/Fault checking/If Action Subsystem/Fault Check (Bulk UVP)/Chart ==
  (default) -> (junction 47)
  (junction 47) -> (junction 50) [order 2]
  (junction 50) -> (junction 52) : {
      | Vbulk_UVP_Threshold=-10;
      | Vbulk_UVP_Flag=1;
      | }
  (junction 47) -> (junction 18) [order 1] : [Soft_Start==0 ]
      | {Vbulk_UVP_Threshold=50;}
  (junction 18) -> (junction 64) [order 1] : [Vbulk < Vbulk_UVP_Threshold]
  (junction 64) -> (junction 76) [order 2] : {
      | Vbulk_UVP_Flag=0;
      | UVPCnt=0;
      | }
  (junction 18) -> (junction 28) [order 2]
  (junction 64) -> (junction 68) [order 1] : [UVPCnt<100]
      | {UVPCnt = UVPCnt + 1;}
  (junction 76) -> (junction 78)
  (junction 52) -> (junction 10)
  (junction 10) -> (junction 38)
  (junction 28) -> (junction 38)
  (junction 68) -> (junction 28)
  (junction 78) -> (junction 68)
  data: VbusRefTemp local =0; Vbulk_UVP_Flag output; Soft_Start input; Vbulk_ADC input; Vbulk_Ref_ADC input; Vbulk input; Vbulk_Ref_ADC_Hard_Value local =0; UVPCnt local =0; Vbulk_UVP_Threshold local double =-10

== stateflow chart CLA_Sample/Calibration,RMS, Fault Protection @5kHz/Relay control/Relay_Control ==
  (default) -> (junction 10)
  (junction 10) -> (junction 37) [order 2]
  (junction 37) -> (junction 40) [order 2]
  (junction 10) -> (junction 12) [order 1] : [Vin_peak_ADC>Relay_TurnON_Threshold_ADC]
  (junction 37) -> (junction 25) [order 1] : [Vin_peak_ADC<(Relay_TurnON_Threshold_ADC-5)]
  (junction 40) -> (junction 42)
  (junction 12) -> (junction 49) [order 2] : %% Relay has started.
  (junction 49) -> (junction 67) [order 1] : [PWM_Turned_on==0]
  (junction 67) -> (junction 79) [order 2]
  (junction 12) -> (junction 19) [order 1] : [Relay_Started==0]
      | {Relay_Start_Count = Relay_Start_Count + 1;}
  (junction 49) -> (junction 73) [order 2]
  (junction 67) -> (junction 68) [order 1] : [Counter_Relay > 400]
      | {
      | PWM_Turned_on=1;
      | Counter_Relay=0;
      | }
  (junction 79) -> (junction 81) : {
      | Counter_Relay = Counter_Relay + 1;
      | PWM_Turned_on=0;
      | }
  (junction 25) -> (junction 27) : [PFC_en==0]
      | {
      | Relay_Started=0;
      | Relay_Start_Count = 0;
      | PWM_Turned_on=0;
      | %% Turn off relay GPIO here
      | }
  (junction 19) -> (junction 54) [order 2]
  (junction 19) -> (junction 21) [order 1] : %%[((Vin_peak_ADC-(Vbulk_ADC_Average/2))<VIN_VBUS_DIFF)]
      | %% Vbulk is within range
  (junction 54) -> (junction 51)
  (junction 21) -> (junction 23) : [Relay_Start_Count > RELAY_START_DELAY]
      | %% waited long enough....
      |
      | {
      | Relay_Start_Count = 0;
      | Relay_Started = 1;
      | Counter_Relay=0;
      | %% Start relay GPIO here
      | }
      |
      | %% Relay started
  (junction 23) -> (junction 51)
  (junction 51) -> (junction 73)
  (junction 73) -> (junction 68)
  (junction 81) -> (junction 68)
  (junction 27) -> (junction 81)
  (junction 42) -> (junction 27)
  data: Vin_peak_ADC input; Relay_TurnON_Threshold_ADC input; RELAY_START_DELAY input; Relay_Start_Count local double =0; PFC_en input; Relay_Started output =0; PWM_Turned_on output double =0; Counter_Relay local =0

== stateflow chart CLA_Sample/Calibration,RMS, Fault Protection @5kHz/Fault checking/If Action Subsystem/PFC_en_update_Phase_A/Chart ==
  note: Local variables
      | VbusRefTemp
      | SoftStartCnt
  note: Verror = Vbulk_Ref_ADC_adjusted - Vbulk_ADC;
  (default) -> (junction 47)
  (junction 47) -> (junction 50) [order 4]
  (junction 47) -> (junction 68) [order 1] : [Vin_OVP_Flag]
  (junction 68) -> (junction 80) : {PFC_en=0;}
  (junction 47) -> (junction 15) [order 2] : [Iin_OCP_Flag]
  (junction 50) -> (junction 52) : {
      | PFC_en=1;
      | PFC_en1=1;
      | }
  (junction 47) -> (junction 5) [order 3] : [Vin_UVP_Flag]
  (junction 80) -> (junction 82)
  (junction 82) -> (junction 84)
  (junction 5) -> (junction 38) : {
      | PFC_en=0;
      | PFC_en1=0;
      | }
  (junction 15) -> (junction 20) : {PFC_en=0;
      | PFC_en1=0;}
  (junction 52) -> (junction 38)
  (junction 20) -> (junction 38)
  (junction 84) -> (junction 20)
  data: Vin_UVP_Flag input; VbusRefTemp local =0; Vin_OVP_Flag input; SoftStartCnt local =0; Vbulk_Ref_ADC_Hard_Value local =0; UVPCnt local =0; PFC_en output; PFC_en1 output; Iin_OCP_Flag input; Iin_OCP_Flag1 local

== stateflow chart CLA_Sample/Calibration,RMS, Fault Protection @5kHz/Calibration/Calibration_Phase_B/Chart1 ==
  note: Add more signals if required.
  (default) -> (junction 4)
  (junction 4) -> (junction 10) [order 1]
  (junction 4) -> (junction 22) [order 3]
  (junction 10) -> (junction 17) : [Calibration_Done==1]
  (junction 4) -> (junction 20) [order 2] : [Local_counter<Counter_for_calibration]
      |
      | {
      |
      | input_signal_1_sum=input_signal_1+input_signal_1_sum;
      | input_signal_2_sum=input_signal_2+input_signal_2_sum;
      | Local_counter = Local_counter + 1;
      |
      | }
  (junction 22) -> (junction 24) : %% Local_counter==Counter_for_calibration
      | %% Meaning that count is completed.
      |
      |
      | {
      | output_signal_1=input_signal_1_sum/Local_counter;
      | output_signal_2=input_signal_2_sum/Local_counter;
      | Calibration_Done=1;
      |
      | Local_counter=0; %% Not required, but do it anyway.
      | }
  (junction 17) -> (junction 20)
  (junction 20) -> (junction 24)
  data: Calibration_Done input; input_signal_1 input; input_signal_2 input; Counter_for_calibration input; Local_counter local double =0; input_signal_1_sum local =0; input_signal_2_sum local =0; output_signal_1 output; output_signal_2 output; Calibration_Done output

== stateflow chart CLA_Sample/Calibration,RMS, Fault Protection @5kHz/Voltage RMS//Averag Calculation/Phase_B/RMS Voltage Calculation_Phase_B/Chart ==
  note: counter > (0.5 / minimum line frequncy) x execution frequency of this loop
      | = [ 1 / (2 x 47 Hz) ] x 5 kHz = 53.191
      | Minimum frequency detection is 47Hz.
      | This can detect the voltage change in ~10.63 ms (max).
  (default) -> (junction 2) : {Vabs=abs(input);}
  (junction 2) -> (junction 81) [order 1] : [Vabs>max_tmp]
  (junction 81) -> (junction 82) : {
      | max_tmp=Vabs;
      | counter=counter+1;
      | timer=timer+1;
      | }
  (junction 2) -> (junction 84) [order 2] : {
      | counter=counter+1;
      | timer=timer+1;
      | }
  (junction 82) -> (junction 84)
  (junction 84) -> (junction 8)
  (junction 8) -> (junction 71) [order 1] : [counter==53]
  (junction 71) -> (junction 72) : {
      | counter=0;
      | Vpeak=max_tmp;
      | Vrms = 0.7071*Vpeak;
      | max_tmp=0;
      | }
  (junction 8) -> (junction 64) [order 2]
  (junction 72) -> (junction 64)
  data: input input double; max_tmp local double =0; counter local double =0; Vpeak output; Vrms output; timer local double =0; Vabs local double =0

== stateflow chart CLA_Sample/Calibration,RMS, Fault Protection @5kHz/Voltage RMS//Averag Calculation/Phase_B/Vin_ADC Averaging_Phase_B/Chart1 ==
  (default) -> (junction 1) : {
      | output_y = b0*input_u + b1*input_z1 - a1*output_z1;
      | input_z1 = input_u;
      | output_z1 = output_y;
      | }
  data: input_z1 local =0; output_z1 local =0; output_y output; input_u input; b0 input; b1 input; a1 input

== stateflow chart CLA_Sample/Calibration,RMS, Fault Protection @5kHz/Fault checking/If Action Subsystem/Phase_B_Fault/Fault Check (Input UVP)_Phase_B/Chart1 ==
  (default) -> (junction 2)
  (junction 2) -> (junction 81) [order 1] : [input > Von_Threshold]
  (junction 81) -> (junction 82) : {
      | Input_UVP_Flag=0;
      | Von_Threshold=8;
      | }
  (junction 2) -> (junction 84) [order 2] : {
      | Input_UVP_Flag=1;
      | Von_Threshold = 12;
      | }
  (junction 82) -> (junction 84)
  data: input input double; Input_UVP_Flag output double =1; Von_Threshold local =12

== stateflow chart CLA_Sample/Calibration,RMS, Fault Protection @5kHz/Fault checking/If Action Subsystem/Phase_B_Fault/Input current_OCP_Phase_B/Chart2 ==
  note: Input_in > 1A, Iin_OCP_Flag=1.
  (default) -> (junction 2)
  (junction 2) -> (junction 81) [order 1] : [input_Iin > OCP_Threshold]
  (junction 81) -> (junction 82) : {Iin_OCP_Flag=1;
      | OCP_Threshold=14;
      | }
  (junction 2) -> (junction 84) [order 2] : {Iin_OCP_Flag=0;
      | OCP_Threshold=15;}
  (junction 82) -> (junction 84)
  data: input_Iin input double; Iin_OCP_Flag output double =1; data local; OCP_Threshold input; OCP_Threshold output

== stateflow chart CLA_Sample/Calibration,RMS, Fault Protection @5kHz/Fault checking/If Action Subsystem/Phase_B_Fault/Fault Check (Input OVP)_Phase_B/Chart1 ==
  (default) -> (junction 2)
  (junction 2) -> (junction 81) [order 1] : [input > Voff_Threshold]
  (junction 81) -> (junction 82) : {
      | Input_OVP_Flag=1;
      | Voff_Threshold=95;
      | }
  (junction 2) -> (junction 84) [order 2] : {
      | Input_OVP_Flag=0;
      | Voff_Threshold = 100;
      | }
  (junction 82) -> (junction 84)
  data: input input double; Input_OVP_Flag output double =0; Voff_Threshold local =100

== stateflow chart CLA_Sample/Calibration,RMS, Fault Protection @5kHz/Fault checking/If Action Subsystem/PFC_en_update_Phase_B/Chart ==
  note: Local variables
      | VbusRefTemp
      | SoftStartCnt
  note: Verror = Vbulk_Ref_ADC_adjusted - Vbulk_ADC;
  (default) -> (junction 47)
  (junction 47) -> (junction 50) [order 4]
  (junction 47) -> (junction 68) [order 1] : [Vin_OVP_Flag]
  (junction 68) -> (junction 80) : {PFC_en=0;}
  (junction 47) -> (junction 15) [order 2] : [Iin_OCP_Flag]
  (junction 50) -> (junction 52) : {
      | PFC_en=1;
      | PFC_en1=1;
      | }
  (junction 47) -> (junction 5) [order 3] : [Vin_UVP_Flag]
  (junction 80) -> (junction 82)
  (junction 82) -> (junction 84)
  (junction 5) -> (junction 38) : {
      | PFC_en=0;
      | PFC_en1=0;
      | }
  (junction 15) -> (junction 20) : {PFC_en=0;
      | PFC_en1=0;}
  (junction 52) -> (junction 38)
  (junction 20) -> (junction 38)
  (junction 84) -> (junction 20)
  data: Vin_UVP_Flag input; VbusRefTemp local =0; Vin_OVP_Flag input; SoftStartCnt local =0; Vbulk_Ref_ADC_Hard_Value local =0; UVPCnt local =0; PFC_en output; PFC_en1 output; Iin_OCP_Flag input; Iin_OCP_Flag1 local

== stateflow chart CLA_Sample/Calibration,RMS, Fault Protection @5kHz/Polarity & Near Zero check/Polarity_Near_zero_Phase_B/Chart ==
  note: 1-> Polarity -> Positive Half cycle
      | 0-> Polarity -> Negative Half cycle
  (default) -> (junction 89) : {Vabs=abs(input);}
  (junction 89) -> (junction 99) [order 1] : [input>Vref]
  (junction 89) -> (junction 103) [order 2] : {Polarity=0;}
  (junction 99) -> (junction 101) : {Polarity=1;}
  (junction 103) -> (junction 142) [order 3]
  (junction 101) -> (junction 103)
  (junction 103) -> (junction 133) [order 1] : [Near_zero==0]
      | {Count = Count+1;}
  (junction 142) -> (junction 146)
  (junction 103) -> (junction 120) [order 2] : [Vabs<VZCD_Gap]
      | {Near_zero=0;}
  (junction 133) -> (junction 120) [order 2]
  (junction 133) -> (junction 136) [order 1] : [Count>10]
      | {Near_zero=1;
      | Count=0;}
  (junction 146) -> (junction 120)
  (junction 136) -> (junction 120)
  data: input input double; Polarity output; Vabs local double =0; Vref input; VZCD_Gap input; Near_zero output double =0; Count local =0
